simulink model "Low_level_Controller"  (R2023a)
settings: Solver=VariableStepAuto  StartTime=0.0  StopTime=10.0  RelTol=1e-3
settings Model: Creator=Artem Sannikov  LastModifiedBy=Artem Sannikov

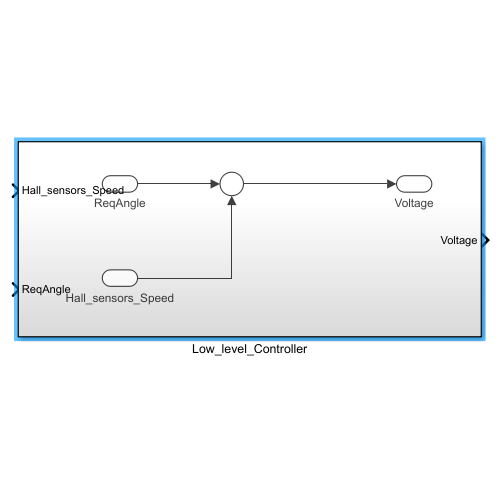
[thumbnail: Simulink's stored preview of the top-level diagram]
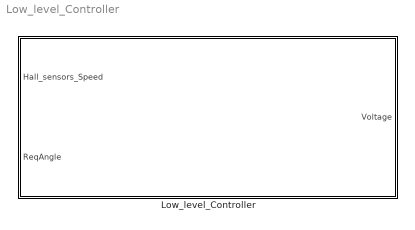
== system Low_level_Controller ==
  Low_level_Controller : Subsystem

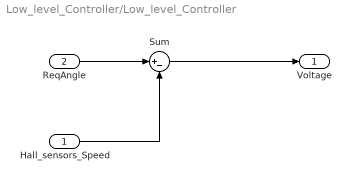
== system Low_level_Controller/Low_level_Controller ==
  Hall_sensors_Speed : Inport
  ReqAngle : Inport  Port=2
  Sum : Sum  Inputs=|+-
  Voltage : Outport
  wires:
  ReqAngle/1 -> Sum/1
  Hall_sensors_Speed/1 -> Sum/2
  Sum/1 -> Voltage/1
